simulink model "FCHEV_sideRadiator"  (R2023a)
settings: Solver=ode23tb  StartTime=0.0  StopTime=20e3  MaxStep=1  RelTol=1e-3
values from neighbouring files (symbols this model uses):
  fc_current = 170    [run_FCHEV_simulations.m]
  mass = 20e3    (= 20000)    [run_BEV_simulations.m]    (also in run_FCHEV_simulations.m)
libraries: component_lib x158, slpidlib x10, simulink x1
(part 1 of 2)
settings Model: Creator=maxjo65  LastModifiedBy=maxjo
settings SolverCC: ZeroCrossControl=DisableAll
settings OptimizationCC: ReuseModelBlockBuffer=off
settings DebuggingCC: UnconnectedInputMsg=warning  UnconnectedOutputMsg=warning  UnconnectedLineMsg=warning
settings ModelReferenceCC: EnableRefExpFcnMdlSchedulingChecks=on
settings RTWCC: DLArmComputeVersion=19.05

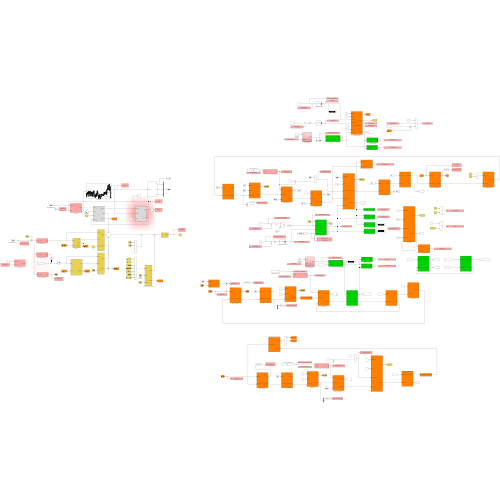
[thumbnail: Simulink's stored preview of the top-level diagram]
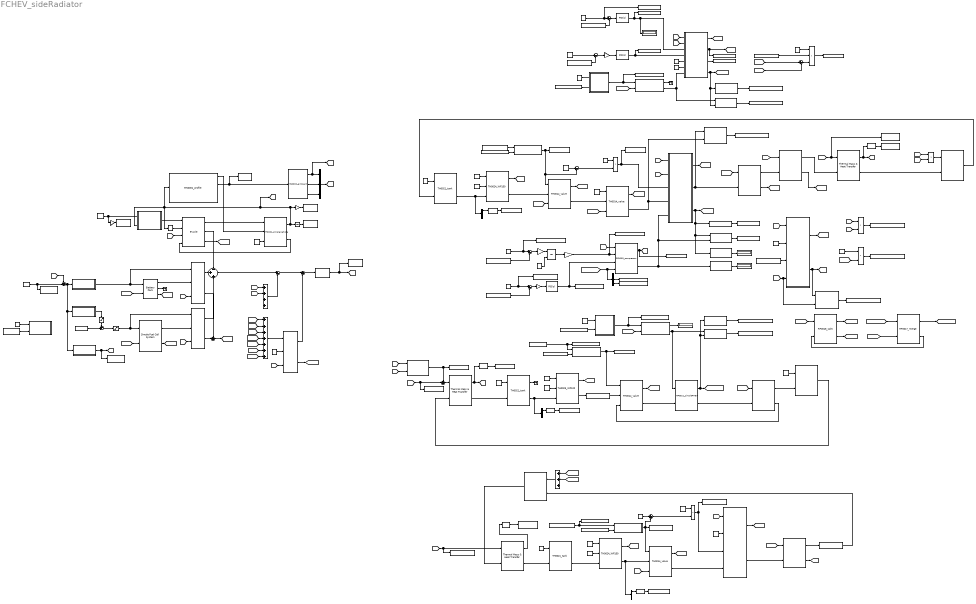
== system FCHEV_sideRadiator ==
  Add Constant{,1..5} (6 alike) : Bias  Bias=-273.15  SaturateOnIntegerOverflow=off
  Add1 : Sum  Inputs=++++
  Add2 : Sum  Inputs=+++++++
  Add3 : Sum  Inputs=+++
  Battery : component_lib/Battery Pack  SOC_0=0.5  Nx=120  Ny=125
  Battery Heater : component_lib/Thermal Systems/TH0015_totalHeatTransfer  T_max=273+100  T_min=273
  Battery Heater1 : component_lib/Thermal Systems/TH0015_totalHeatTransfer  T_max=273+100  T_min=273
  Battery Thermal Mass : component_lib/Thermal Mass & Heat Transfer  n=100  d=10e-3  L=4  m=120 * 125 * 0.048  cp=1040  T_0=273 + 26
  Bus Voltage Control 1 : Subsystem
  "Bus Voltage Control 2 " : Subsystem
  Bus Voltage Control 3 : Subsystem
  Bus Voltage Reference [V] : Constant  Value=700
  Cabin Airflow Controller : slpidlib/PID Controller  Controller=PID  Form=Parallel  TimeDomain=Continuous-time  UseExternalTs=off  SampleTime=-1  IntegratorMethod=Forward Euler  FilterMethod=Forward Euler  ControllerParametersSource=internal  P=1  I=1e-1  UseKiTs=off  D=0  N=100  UseFilter=on  TunerSelectOption=Transfer Function Based (PID Tuner App)  InitialConditionSource=internal  InitialConditionForIntegrator=0.5  InitialConditionForFilter=0.5  DifferentiatorICPrevScaledInput=0  ExternalReset=none  TrackingMode=off  Kt=1  LimitOutput=on  SatLimitsSource=internal  UpperSaturationLimit=0.99  LowerSaturationLimit=0.01  LinearizeAsGain=on  AntiWindupMode=clamping  Kb=1  LimitIntegrator=off  UpperIntegratorSaturationLimit=inf  LowerIntegratorSaturationLimit=-inf  POutMin=[]  POutMax=[]  IOutMin=[]  IOutMax=[]  DOutMin=[]  DOutMax=[]  NOutMin=[]  NOutMax=[]  SumOutMin=[]  SumOutMax=[]  SaturationOutMin=[]  SaturationOutMax=[]  PParamMin=[]  PParamMax=[]  IParamMin=[]  IParamMax=[]  DParamMin=[]  DParamMax=[]  NParamMin=[]  NParamMax=[]  KbParamMin=[]  KbParamMax=[]  KtParamMin=[]  KtParamMax=[]  KbOutMin=[]  KbOutMax=[]  KtOutMin=[]  KtOutMax=[]  IntegratorOutMin=[]  IntegratorOutMax=[]  FilterOutMin=[]  FilterOutMax=[]  SumI1OutMin=[]  SumI1OutMax=[]  SumI2OutMin=[]  SumI2OutMax=[]  SumI3OutMin=[]  SumI3OutMax=[]  SumI4OutMin=[]  SumI4OutMax=[]  SumDOutMin=[]  SumDOutMax=[]  DifferentiatorOutMin=[]  DifferentiatorOutMax=[]  FilterDiffOutCoefMin=[]  FilterDiffOutCoefMax=[]  ReciprocalOutMin=[]  ReciprocalOutMax=[]  SumDenOutMin=[]  SumDenOutMax=[]  SumNumOutMin=[]  SumNumOutMax=[]  DivideOutMin=[]  DivideOutMax=[]  UdiffTsProdOutMin=[]  UdiffTsProdOutMax=[]  NTsProdOutMin=[]  NTsProdOutMax=[]  UintegralTsProdOutMin=[]  UintegralTsProdOutMax=[]  UngainTsProdOutMin=[]  UngainTsProdOutMax=[]  ClampingZeroOutDataTypeStr=Inherit: Inherit via back propagation  ClampingZeroOutMin=[]  ClampingZeroOutMax=[]  FilterDenConstantOutDataTypeStr=Inherit: Inherit via back propagation  FilterDenConstantOutMin=[]  FilterDenConstantOutMax=[]  PCopyOutDataTypeStr=Inherit: Inherit via back propagation  PCopyOutMin=[]  PCopyOutMax=[]  NCopyOutDataTypeStr=Inherit: Inherit via back propagation  NCopyOutMin=[]  NCopyOutMax=[]  IntegratorContinuousStateAttributes=''  IntegratorStateMustResolveToSignalObject=off  IntegratorRTWStateStorageClass=Auto  FilterContinuousStateAttributes=''  FilterStateMustResolveToSignalObject=off  FilterRTWStateStorageClass=Auto  ParallelPVariant=InternalParameters  IdealPVariant=Disabled  IVariant=InternalParameters  DVariant=InternalParameters  IntegratorVariant=Continuous  SatVariant=Enabled  AWVariant=ContClampingParallel  PCopyVariant=Disabled  TRVariant=Disabled  FdbkBlocksVariant=Forward  IdealPFdbkVariant=Disabled  SatFdbkVariant=Disabled  DerivativeFilterVariant=ContFilter  NVariant=InternalParameters  NCopyVariant=Disabled  FilterICVariant=InternalICsFilter  IntegratorICVariant=InternalICs  ExternalResetVariant=Disabled  TRSumVariant=Passthrough  SumFdbkVariant=Disabled  SumVariant=Sum_PID  TsampFilterVariant=InternalTs  TsampNgainVariant=Passthrough  TsampIntegralVariant=Disabled_SignalSpec  ExternalSaturationOutDataTypeStr=Inherit: Same as second input
  Cabin Temperature Controller : slpidlib/PID Controller  Controller=PID  Form=Parallel  TimeDomain=Continuous-time  UseExternalTs=off  SampleTime=-1  IntegratorMethod=Forward Euler  FilterMethod=Forward Euler  ControllerParametersSource=internal  P=1e-1  I=1e-2  UseKiTs=off  D=0  N=100  UseFilter=on  TunerSelectOption=Transfer Function Based (PID Tuner App)  InitialConditionSource=internal  InitialConditionForIntegrator=0.5  InitialConditionForFilter=0.5  DifferentiatorICPrevScaledInput=0  ExternalReset=none  TrackingMode=off  Kt=1  LimitOutput=on  SatLimitsSource=internal  UpperSaturationLimit=0.99  LowerSaturationLimit=0.01  LinearizeAsGain=on  AntiWindupMode=clamping  Kb=1  LimitIntegrator=off  UpperIntegratorSaturationLimit=inf  LowerIntegratorSaturationLimit=-inf  POutMin=[]  POutMax=[]  IOutMin=[]  IOutMax=[]  DOutMin=[]  DOutMax=[]  NOutMin=[]  NOutMax=[]  SumOutMin=[]  SumOutMax=[]  SaturationOutMin=[]  SaturationOutMax=[]  PParamMin=[]  PParamMax=[]  IParamMin=[]  IParamMax=[]  DParamMin=[]  DParamMax=[]  NParamMin=[]  NParamMax=[]  KbParamMin=[]  KbParamMax=[]  KtParamMin=[]  KtParamMax=[]  KbOutMin=[]  KbOutMax=[]  KtOutMin=[]  KtOutMax=[]  IntegratorOutMin=[]  IntegratorOutMax=[]  FilterOutMin=[]  FilterOutMax=[]  SumI1OutMin=[]  SumI1OutMax=[]  SumI2OutMin=[]  SumI2OutMax=[]  SumI3OutMin=[]  SumI3OutMax=[]  SumI4OutMin=[]  SumI4OutMax=[]  SumDOutMin=[]  SumDOutMax=[]  DifferentiatorOutMin=[]  DifferentiatorOutMax=[]  FilterDiffOutCoefMin=[]  FilterDiffOutCoefMax=[]  ReciprocalOutMin=[]  ReciprocalOutMax=[]  SumDenOutMin=[]  SumDenOutMax=[]  SumNumOutMin=[]  SumNumOutMax=[]  DivideOutMin=[]  DivideOutMax=[]  UdiffTsProdOutMin=[]  UdiffTsProdOutMax=[]  NTsProdOutMin=[]  NTsProdOutMax=[]  UintegralTsProdOutMin=[]  UintegralTsProdOutMax=[]  UngainTsProdOutMin=[]  UngainTsProdOutMax=[]  ClampingZeroOutDataTypeStr=Inherit: Inherit via back propagation  ClampingZeroOutMin=[]  ClampingZeroOutMax=[]  FilterDenConstantOutDataTypeStr=Inherit: Inherit via back propagation  FilterDenConstantOutMin=[]  FilterDenConstantOutMax=[]  PCopyOutDataTypeStr=Inherit: Inherit via back propagation  PCopyOutMin=[]  PCopyOutMax=[]  NCopyOutDataTypeStr=Inherit: Inherit via back propagation  NCopyOutMin=[]  NCopyOutMax=[]  IntegratorContinuousStateAttributes=''  IntegratorStateMustResolveToSignalObject=off  IntegratorRTWStateStorageClass=Auto  FilterContinuousStateAttributes=''  FilterStateMustResolveToSignalObject=off  FilterRTWStateStorageClass=Auto  ParallelPVariant=InternalParameters  IdealPVariant=Disabled  IVariant=InternalParameters  DVariant=InternalParameters  IntegratorVariant=Continuous  SatVariant=Enabled  AWVariant=ContClampingParallel  PCopyVariant=Disabled  TRVariant=Disabled  FdbkBlocksVariant=Forward  IdealPFdbkVariant=Disabled  SatFdbkVariant=Disabled  DerivativeFilterVariant=ContFilter  NVariant=InternalParameters  NCopyVariant=Disabled  FilterICVariant=InternalICsFilter  IntegratorICVariant=InternalICs  ExternalResetVariant=Disabled  TRSumVariant=Passthrough  SumFdbkVariant=Disabled  SumVariant=Sum_PID  TsampFilterVariant=InternalTs  TsampNgainVariant=Passthrough  TsampIntegralVariant=Disabled_SignalSpec  ExternalSaturationOutDataTypeStr=Inherit: Same as second input
  Cabin with Evaporator : Subsystem
  Calculate Superheat1 : component_lib/Thermal Systems/RF0010_calculateSuperHeat
  Calculate Superheat2 : component_lib/Thermal Systems/RF0010_calculateSuperHeat
  Chassi : component_lib/Powertrain/PT0001_simpleVehicle  m=mass  r_w=0.5  A_f=10  C_d=0.5  rho_air=1.225  c_r0=0.0060  c_r1=2.3e-7  gain=600  v0=80/3.6  x0=0
  Chiller Bypass : component_lib/Thermal Systems/TH0014_valve  d=10e-2  dr=5e-2  C_d=0.9
  Compressor Speed Controller : slpidlib/PID Controller  Controller=PID  Form=Parallel  TimeDomain=Continuous-time  UseExternalTs=off  SampleTime=-1  IntegratorMethod=Forward Euler  FilterMethod=Forward Euler  ControllerParametersSource=internal  P=1e2  I=1e1  UseKiTs=off  D=0  N=100  UseFilter=on  TunerSelectOption=Transfer Function Based (PID Tuner App)  InitialConditionSource=internal  InitialConditionForIntegrator=2000  InitialConditionForFilter=2000  DifferentiatorICPrevScaledInput=0  ExternalReset=none  TrackingMode=off  Kt=1  LimitOutput=on  SatLimitsSource=internal  UpperSaturationLimit=5000  LowerSaturationLimit=100  LinearizeAsGain=on  AntiWindupMode=clamping  Kb=1  LimitIntegrator=off  UpperIntegratorSaturationLimit=inf  LowerIntegratorSaturationLimit=-inf  POutMin=[]  POutMax=[]  IOutMin=[]  IOutMax=[]  DOutMin=[]  DOutMax=[]  NOutMin=[]  NOutMax=[]  SumOutMin=[]  SumOutMax=[]  SaturationOutMin=[]  SaturationOutMax=[]  PParamMin=[]  PParamMax=[]  IParamMin=[]  IParamMax=[]  DParamMin=[]  DParamMax=[]  NParamMin=[]  NParamMax=[]  KbParamMin=[]  KbParamMax=[]  KtParamMin=[]  KtParamMax=[]  KbOutMin=[]  KbOutMax=[]  KtOutMin=[]  KtOutMax=[]  IntegratorOutMin=[]  IntegratorOutMax=[]  FilterOutMin=[]  FilterOutMax=[]  SumI1OutMin=[]  SumI1OutMax=[]  SumI2OutMin=[]  SumI2OutMax=[]  SumI3OutMin=[]  SumI3OutMax=[]  SumI4OutMin=[]  SumI4OutMax=[]  SumDOutMin=[]  SumDOutMax=[]  DifferentiatorOutMin=[]  DifferentiatorOutMax=[]  FilterDiffOutCoefMin=[]  FilterDiffOutCoefMax=[]  ReciprocalOutMin=[]  ReciprocalOutMax=[]  SumDenOutMin=[]  SumDenOutMax=[]  SumNumOutMin=[]  SumNumOutMax=[]  DivideOutMin=[]  DivideOutMax=[]  UdiffTsProdOutMin=[]  UdiffTsProdOutMax=[]  NTsProdOutMin=[]  NTsProdOutMax=[]  UintegralTsProdOutMin=[]  UintegralTsProdOutMax=[]  UngainTsProdOutMin=[]  UngainTsProdOutMax=[]  ClampingZeroOutDataTypeStr=Inherit: Inherit via back propagation  ClampingZeroOutMin=[]  ClampingZeroOutMax=[]  FilterDenConstantOutDataTypeStr=Inherit: Inherit via back propagation  FilterDenConstantOutMin=[]  FilterDenConstantOutMax=[]  PCopyOutDataTypeStr=Inherit: Inherit via back propagation  PCopyOutMin=[]  PCopyOutMax=[]  NCopyOutDataTypeStr=Inherit: Inherit via back propagation  NCopyOutMin=[]  NCopyOutMax=[]  IntegratorContinuousStateAttributes=''  IntegratorStateMustResolveToSignalObject=off  IntegratorRTWStateStorageClass=Auto  FilterContinuousStateAttributes=''  FilterStateMustResolveToSignalObject=off  FilterRTWStateStorageClass=Auto  ParallelPVariant=InternalParameters  IdealPVariant=Disabled  IVariant=InternalParameters  DVariant=InternalParameters  IntegratorVariant=Continuous  SatVariant=Enabled  AWVariant=ContClampingParallel  PCopyVariant=Disabled  TRVariant=Disabled  FdbkBlocksVariant=Forward  IdealPFdbkVariant=Disabled  SatFdbkVariant=Disabled  DerivativeFilterVariant=ContFilter  NVariant=InternalParameters  NCopyVariant=Disabled  FilterICVariant=InternalICsFilter  IntegratorICVariant=InternalICs  ExternalResetVariant=Disabled  TRSumVariant=Passthrough  SumFdbkVariant=Disabled  SumVariant=Sum_PID  TsampFilterVariant=InternalTs  TsampNgainVariant=Passthrough  TsampIntegralVariant=Disabled_SignalSpec  ExternalSaturationOutDataTypeStr=Inherit: Same as second input
  Constant : Constant  Value=0.3
  Constant{1,11,13,19,27} (5 alike) : Constant  Value=0
  Constant{6,8,10,17} (4 alike) : Constant  Value=24
  Constant12 : Constant  Value=23
  Constant14 : Constant  Value=0.1
  Constant15 : Constant  Value=2e5
  Constant16 : Constant  Value=4000
  Constant{2,5,18,21,26} (5 alike) : Constant  Value=3000
  Constant20 : Constant  Value=22.5
  Constant23 : Constant  Value=10
  Constant24 : Constant  Value=15
  Constant25 : Constant
  Constant28 : Constant
  Constant3 : Constant  Value=0.5
  Constant4 : Constant  Value=2e5
  Constant7 : Constant  Value=2e5
  Constant9 : Constant  Value=fc_current
  DC/DC - Low level converter : component_lib/Electrochemistry/EL0008_dcdcConverter  eta_up=0.98  eta_down=0.98
  DC/DC Converter : component_lib/Electrochemistry/EL0008_dcdcConverter  eta_up=0.99  eta_down=0.99
  DC/DC Converter1 : component_lib/Electrochemistry/EL0008_dcdcConverter  eta_up=0.99  eta_down=0.99
  Demux{,1..3} (4 alike) : Demux  Outputs=3
  Display{,1..3} (4 alike) : Display
  Fuel Cell Thermal Mass : component_lib/Thermal Mass & Heat Transfer  n=375*2*20  d=2e-3  L=50e-2  m=72  cp=420  T_0=273 + 80
  Gain : Gain  Gain=3.6
  Gain1 : Gain  Gain=3.6
  Gain2 : Gain  Gain=-1
  Gain3 : Gain  Gain=-1
  Gain4 : Gain  Gain=1e5
  Gain5 : Gain  Gain=1e-1
  Gear selector : Relay  OnSwitchValue=22  OffSwitchValue=21.5  OnOutputValue=4  OffOutputValue=3
  Integrator : Integrator
  Integrator1 : Integrator  InitialConditionSource=external  LimitOutput=on  UpperSaturationLimit=30  LowerSaturationLimit=8
  Low Voltage Bus Level : Constant  Value=24
  MN0002_ambient : component_lib/Mission/MN0002_ambient  p_0=1.01e5  T_0=T_amb  RH_0=0.2
  Motor Heat Transfer : component_lib/Thermal Mass & Heat Transfer  n=100*3  d=5e-3  L=30e-2  m=200  cp=420  T_0=273 + 70
  Motor Temperature Reference : Constant  Value=70
  Motor and Gearbox : component_lib/E-Axle  n=4  V_nom=700
  Mux : Mux  Inputs=3
  Power Electronics Heat Transfer : component_lib/Thermal Systems/TH0015_totalHeatTransfer  T_max=273+100  T_min=273
  Product : Product  Inputs=***
  Product{1..5} (5 alike) : Product
  RF0003_compressor : component_lib/Thermal Systems/RF0003_compressor  V_disp=0.00017  N_ref=2000  t_c=1  W0=25e-3
  RF0011_calculateSubCool : component_lib/Thermal Systems/RF0011_calculateSubCool
  RF0013_calculateHeatflow1 : component_lib/Thermal Systems/RF0013_calculateHeatflow
  RF0013_calculateHeatflow2 : component_lib/Thermal Systems/RF0013_calculateHeatflow
  RF0013_calculateHeatflow3 : component_lib/Thermal Systems/RF0013_calculateHeatflow
  RF0016_split : component_lib/Thermal Systems/RF0016_split
  RF0017_merge : component_lib/Thermal Systems/RF0017_merge  V=1e-3
  RF0018_calculateTemperature : component_lib/Thermal Systems/RF0018_calculateTemperature
  RF0018_calculateTemperature1 : component_lib/Thermal Systems/RF0018_calculateTemperature
  RF0021_simplePHEX : component_lib/Thermal Systems/RF0021_simplePHEX  N_ch=10  L=180e-3  B=65e-3  H=2e-3  t=0.3e-3  D_h=2.61e-3
  RF0022_simpleExpansionValve : component_lib/Thermal Systems/RF0022_simpleExpansionValve  D=4*1.8e-3  p_min=100e3  C=0.3
  RF0022_simpleExpansionValve1 : component_lib/Thermal Systems/RF0022_simpleExpansionValve  D=4*1.8e-3  p_min=100e3  C=0.3
  Radiator & Condenser Assembly : Subsystem
  Radiator Bypass Valve : component_lib/Thermal Systems/TH0014_valve  d=10e-2  dr=5e-2  C_d=0.9
  Radiator Bypass Valve1 : component_lib/Thermal Systems/TH0014_valve  d=10e-2  dr=5e-2  C_d=0.9
  Road Profile : component_lib/Mission/MN0001_profile  profile=Sodertalje_Norrkoping.mat  x0=0  N_lookahead=100
  SC0002_signalRead : component_lib/Data & Control/SC0002_signalRead  SigName=velocity
  SC0002_signalRead1 : component_lib/Data & Control/SC0002_signalRead  SigName=condenserCooling
  SC0002_signalRead10 : component_lib/Data & Control/SC0002_signalRead  SigName=condenserSubcool
  SC0002_signalRead11 : component_lib/Data & Control/SC0002_signalRead  SigName=chillerBypassValve
  SC0002_signalRead12 : component_lib/Data & Control/SC0002_signalRead  SigName=batteryTemperatureReference
  SC0002_signalRead13 : component_lib/Data & Control/SC0002_signalRead  SigName=cabinFreshAirFlowReference
  SC0002_signalRead14 : component_lib/Data & Control/SC0002_signalRead  SigName=intakeFlap
  SC0002_signalRead15 : component_lib/Data & Control/SC0002_signalRead  SigName=cabinFreshAirFlow
  SC0002_signalRead16 : component_lib/Data & Control/SC0002_signalRead  SigName=batteryConvection
  SC0002_signalRead17 : component_lib/Data & Control/SC0002_signalRead  SigName=batteryCoolantTemperature
  SC0002_signalRead18 : component_lib/Data & Control/SC0002_signalRead  SigName=fuelCellTemperature
  SC0002_signalRead19 : component_lib/Data & Control/SC0002_signalRead  SigName=radiatorBypassValve
  SC0002_signalRead2 : component_lib/Data & Control/SC0002_signalRead  SigName=altitude
  SC0002_signalRead20 : component_lib/Data & Control/SC0002_signalRead  SigName=evaporatorExpansionValve
  SC0002_signalRead21 : component_lib/Data & Control/SC0002_signalRead  SigName=mainRadiatorFanSpeed
  SC0002_signalRead22 : component_lib/Data & Control/SC0002_signalRead  SigName=batteryTemperature
  SC0002_signalRead23 : component_lib/Data & Control/SC0002_signalRead  SigName=evaporatorSuperheat
  SC0002_signalRead24 : component_lib/Data & Control/SC0002_signalRead  SigName=chillerCooling
  SC0002_signalRead25 : component_lib/Data & Control/SC0002_signalRead  SigName=motorTemperature
  SC0002_signalRead26 : component_lib/Data & Control/SC0002_signalRead  SigName=sideRadiatorBypassValve
  SC0002_signalRead27 : component_lib/Data & Control/SC0002_signalRead  SigName=motorCoolantTemperatureReference
  SC0002_signalRead28 : component_lib/Data & Control/SC0002_signalRead  SigName=chillerSuperheat
  SC0002_signalRead29 : component_lib/Data & Control/SC0002_signalRead  SigName=cabinFanCurrent
  SC0002_signalRead3 : component_lib/Data & Control/SC0002_signalRead  SigName=velocityReference
  SC0002_signalRead30 : component_lib/Data & Control/SC0002_signalRead  SigName=chillerExpansionValve
  SC0002_signalRead31 : component_lib/Data & Control/SC0002_signalRead  SigName=evaporatorCooling
  SC0002_signalRead33 : component_lib/Data & Control/SC0002_signalRead  SigName=evaporatorFlap
  SC0002_signalRead34 : component_lib/Data & Control/SC0002_signalRead  SigName=compressorCurrent
  SC0002_signalRead35 : component_lib/Data & Control/SC0002_signalRead  SigName=condenserPressure
  SC0002_signalRead36 : component_lib/Data & Control/SC0002_signalRead  SigName=fuelCellLosses
  SC0002_signalRead37 : component_lib/Data & Control/SC0002_signalRead  SigName=fanPower
  SC0002_signalRead38 : component_lib/Data & Control/SC0002_signalRead  SigName=evaporatorPressure
  SC0002_signalRead39 : component_lib/Data & Control/SC0002_signalRead  SigName=compressorFlow
  SC0002_signalRead4 : component_lib/Data & Control/SC0002_signalRead  SigName=busVoltage
  SC0002_signalRead40 : component_lib/Data & Control/SC0002_signalRead  SigName=compressorPower
  SC0002_signalRead41 : component_lib/Data & Control/SC0002_signalRead  SigName=batteryLosses
  SC0002_signalRead42 : component_lib/Data & Control/SC0002_signalRead  SigName=cabinIntakeHeat
  SC0002_signalRead43 : component_lib/Data & Control/SC0002_signalRead  SigName=condenserSubcoolReference
  SC0002_signalRead44 : component_lib/Data & Control/SC0002_signalRead  SigName=sideRadiatorCooling
  SC0002_signalRead45 : component_lib/Data & Control/SC0002_signalRead  SigName=mainRadiatorCooling
  SC0002_signalRead46 : component_lib/Data & Control/SC0002_signalRead  SigName=motorLosses
  SC0002_signalRead47 : component_lib/Data & Control/SC0002_signalRead  SigName=motorRadiatorFanSpeed
  SC0002_signalRead48 : component_lib/Data & Control/SC0002_signalRead  SigName=compressorSpeed
  SC0002_signalRead49 : component_lib/Data & Control/SC0002_signalRead  SigName=cabinTemperatureReference
  SC0002_signalRead5 : component_lib/Data & Control/SC0002_signalRead  SigName=distance
  SC0002_signalRead6 : component_lib/Data & Control/SC0002_signalRead  SigName=busVoltageReference
  SC0002_signalRead7 : component_lib/Data & Control/SC0002_signalRead  SigName=burnoffCurrent
  SC0002_signalRead8 : component_lib/Data & Control/SC0002_signalRead  SigName=fuelCellCoolantTemperature
  SC0002_signalRead9 : component_lib/Data & Control/SC0002_signalRead  SigName=motorCoolantTemperature
  SC0003_signalWrite : component_lib/Data & Control/SC0003_signalWrite  SigName=stateOfCharge
  SC0003_signalWrite1 : component_lib/Data & Control/SC0003_signalWrite  SigName=batteryCoolantTemperature
  SC0003_signalWrite10 : component_lib/Data & Control/SC0003_signalWrite  SigName=mainRadiatorFanSpeed
  SC0003_signalWrite15 : component_lib/Data & Control/SC0003_signalWrite  SigName=cabinFreshAirFlow
  SC0003_signalWrite2 : component_lib/Data & Control/SC0003_signalWrite  SigName=cabinFreshAirFlow
  SC0003_signalWrite3 : component_lib/Data & Control/SC0003_signalWrite  SigName=fuelCellTemperature
  SC0003_signalWrite4 : component_lib/Data & Control/SC0003_signalWrite  SigName=motorCoolantTemperature
  SC0003_signalWrite5 : component_lib/Data & Control/SC0003_signalWrite  SigName=chillerSuperheat
  SC0003_signalWrite6 : component_lib/Data & Control/SC0003_signalWrite  SigName=evaporatorSuperheat
  SC0003_signalWrite7 : component_lib/Data & Control/SC0003_signalWrite  SigName=cabinTemperature
  SC0003_signalWrite8 : component_lib/Data & Control/SC0003_signalWrite  SigName=cabinTemperature
  SC0003_signalWrite9 : component_lib/Data & Control/SC0003_signalWrite  SigName=condenserSubcool
  SOC-reference : Subsystem
  Saturation : Saturate  UpperLimit=500  LowerLimit=20
  Saturation1 : Saturate  UpperLimit=0  LowerLimit=-inf
  Side Radiator Valve : component_lib/Thermal Systems/TH0014_valve  d=10e-2  dr=5e-2  C_d=0.9
  Side radiator : Subsystem  mask{HtH=0.5, StS=0.5}
      mask prompts: HtH "Header to header [m]"; StS "Sideplate to sideplate [m]"
  Simple Fuel Cell System : component_lib/Simple Fuel Cell System  n_st=2  n=400
  Single Air Stream Heat Exchanger : Subsystem  mask{HtH=0.5, StS=0.5}
      mask prompts: HtH "Header to header [m]"; StS "Sideplate to sideplate [m]"
  Speed control : Subsystem
  Speed reference [m/s] : Constant  Value=80/3.6
  Subsystem1 : Subsystem
  Subsystem2 : Subsystem
  Subsystem4 : Subsystem
  Sum : Sum  Inputs=-++
  Sum1 : Sum  Inputs=-+|
  Sum{3..4,7..13} (9 alike) : Sum  Inputs=|+-
  Sum2 : Sum  Inputs=++|
  Sum5 : Sum  Inputs=++|
  Sum6 : Sum  Inputs=++|
  Super Capacitor : component_lib/Electrochemistry/EL0010_superCapacitor  C=1  V_bus0=700
  Superheat Control : Subsystem
  Superheat Control1 : Subsystem
  Superheating Reference : Constant  Value=5
  Superheating Reference1 : Constant  Value=5
  TH0006_flowConfluence{1..4} (4 alike) : component_lib/Thermal Systems/TH0006_flowConfluence  gain=0.01
  TH0011_pipe1 : component_lib/Thermal Systems/TH0011_pipe  d=19e-3  L=2  e=0.006e-3  T_0=273 + 20
  TH0011_pipe2 : component_lib/Thermal Systems/TH0011_pipe  d=32e-3  L=2  e=0.006e-3  T_0=273 + 20
  TH0016_calculateHeatflow : component_lib/Thermal Systems/TH0016_calculateHeatflow
  TH0016_calculateHeatflow1 : component_lib/Thermal Systems/TH0016_calculateHeatflow
  TH0021_tank : component_lib/Thermal Systems/TH0021_tank  V=5e-3  T0=273.15 + 25
  TH0021_tank1 : component_lib/Thermal Systems/TH0021_tank  V=5e-3  T0=273.15 + 80
  TH0021_tank2 : component_lib/Thermal Systems/TH0021_tank  V=5e-3  T0=273.15 + 70
  TH0023_WP120 : component_lib/Thermal Systems/TH0023_WP120  SystemSampleTime=-1  VariantActivationTime=update diagram  Latency=0  AutoFrameSizeCalculation=off
  TH0024_WP1 : component_lib/Thermal Systems/TH0024_WP150  n=2
      settings: LibrarySourceBlock=component_lib/Thermal Systems/TH0023_WP120
  TH0024_WP150 : component_lib/Thermal Systems/TH0024_WP150  n=2
      settings: LibrarySourceBlock=component_lib/Thermal Systems/TH0023_WP120
  TH0030_batteryPackConvection : component_lib/Thermal Systems/TH0030_batteryPackConvection  A=2*10  h=8
  Temperature Reference : Constant  Value=80
  Temperature Reference2 : Constant  Value=25
  Terminator : Terminator
  Terminator2 : Terminator
  Terminator3 : Terminator
  cp_air : Constant  Value=1e3
  wires:
  Motor and Gearbox/1 -> Chassi/1
  Chassi/2 -> Motor and Gearbox/4
  Road Profile/1 -> Chassi/2
  Chassi/1 -> Integrator/1, Gain/1, [v], Speed control/2(v [m/s]), Road Profile/1, Gear selector/1
  Speed reference [m/s]/1 -> Gain1/1, Speed control/1(v_ref [m/s])
  Speed control/1(Tq_sig [-]) -> Motor and Gearbox/1
  Gear selector/1 -> Motor and Gearbox/2
  Integrator/1 -> SC0002_signalRead5/1
  Gain/1 -> SC0002_signalRead/1
  Road Profile/2 -> MN0002_ambient/1, SC0002_signalRead2/1
  Gain1/1 -> SC0002_signalRead3/1
  Super Capacitor/1 -> SC0002_signalRead4/1, [V_bus]
  Constant1/1 -> Chassi/3
  Battery/1 -> DC/DC Converter/2
  DC/DC Converter/1 -> Sum/2
  Motor and Gearbox/2 -> Sum/1
  Bus Voltage Control 1/1(I_bat [-]) -> DC/DC Converter/1, Battery/1
  DC/DC Converter1/1 -> Sum/3
  Bus Voltage Reference [V]/1 -> Sum1/2, SC0002_signalRead6/1
  Constant3/1 -> SOC-reference/1(SOC_ref [-])
  SC0003_signalWrite/1 -> SOC-reference/2(SOC [-])
  Sum1/1 -> Bus Voltage Control 3/1(V_ref - V_bus [V]), "Bus Voltage Control 2 "/1(V_ref - V_bus [V]), Bus Voltage Control 1/1(V_ref - V_bus [V])
  Sum2/1 -> Saturation/1
  Sum/1 -> Sum3/1
  Bus Voltage Control 3/1(I_bf [A]) -> SC0002_signalRead7/1, [I_bf]
  Simple Fuel Cell System/1 -> DC/DC Converter1/2
  Sum3/1 -> Sum4/1
  Saturation/1 -> DC/DC Converter1/1, Simple Fuel Cell System/1
  [T_bat] -> Battery/2
  Sum4/1 -> Super Capacitor/1
  Low Voltage Bus Level/1 -> DC/DC - Low level converter/2
  DC/DC - Low level converter/1 -> Sum4/2
  DC/DC - Low level converter/2 -> [Q_LVDCDC]
  [I_cabFan] -> Add2/1
  [I_batPump] -> Add2/2
  [V_bus] -> DC/DC - Low level converter/3
  [I_radPump] -> Add2/3
  Add2/1 -> DC/DC - Low level converter/1
  Sum5/1 -> Battery Thermal Mass/1
  [T_bat] -> TH0030_batteryPackConvection/2
  TH0021_tank/2 -> Demux/1, TH0023_WP120/3
  TH0023_WP120/1 -> [I_batPump]
  Add Constant1/1 -> SC0002_signalRead17/1
  Constant6/1 -> TH0023_WP120/1
  TH0021_tank/1 -> Terminator3/1
  Add Constant/1 -> SC0002_signalRead22/1
  RF0021_simplePHEX/1 -> Calculate Superheat1/1, RF0013_calculateHeatflow1/2, [RF_CHILLER_OUT]
  TH0011_pipe1/1 -> Chiller Bypass/2
  TH0030_batteryPackConvection/1 -> Sum5/1, SC0002_signalRead16/1
  RF0022_simpleExpansionValve/2 -> RF0021_simplePHEX/1, RF0013_calculateHeatflow1/1
  Constant5/1 -> TH0023_WP120/2
  Demux/1 -> Add Constant1/1
  Constant4/1 -> TH0021_tank/1
  RF0013_calculateHeatflow1/1 -> SC0002_signalRead24/1
  Battery Thermal Mass/2 -> TH0021_tank/2
  Battery Thermal Mass/1 -> [T_bat], Add Constant/1
  TH0023_WP120/2 -> TH0011_pipe1/1
  [T_amb] -> TH0030_batteryPackConvection/1
  MN0002_ambient/2 -> Mux/2
  MN0002_ambient/3 -> Mux/3
  MN0002_ambient/1 -> [T_amb], Mux/1
  Mux/1 -> [amb]
  Simple Fuel Cell System/2 -> [Q_fc]
  Battery/3 -> [Q_bat]
  Motor and Gearbox/3 -> [Q_em]
  DC/DC Converter1/2 -> Sum6/2
  Sum6/1 -> [Q_HVDCDC]
  DC/DC Converter/2 -> Sum6/1
  [T_fc] -> Simple Fuel Cell System/2
  [V_bus] -> Motor and Gearbox/3
  [V_bus] -> Sum1/1
  [V_bus] -> DC/DC Converter/3
  [V_bus] -> DC/DC Converter1/3
  Superheating Reference/1 -> Superheat Control/1(T_ref [K])
  [RF_CHILLER_IN] -> RF0022_simpleExpansionValve/2
  SC0003_signalWrite5/1 -> Superheat Control/2(T_sup [K])
  Superheat Control/1(EXV [-]) -> RF0022_simpleExpansionValve/1, SC0002_signalRead30/1
  RF0022_simpleExpansionValve/1 -> Display/1
  Radiator Bypass Valve/1 -> [CL1]
  Battery Heater1/1 -> TH0021_tank1/2
  Temperature Reference/1 -> Subsystem1/1(T_ref [K])
  Radiator & Condenser Assembly/2(CL: (T2,p2,W2)) -> TH0016_calculateHeatflow1/1, TH0006_flowConfluence1/2
  Constant7/1 -> TH0021_tank1/1
  [Q_fc] -> SC0002_signalRead36/1, Fuel Cell Thermal Mass/1
  SC0003_signalWrite3/1 -> Subsystem1/2(T_fc [K])
  Radiator Bypass Valve/2 -> Side Radiator Valve/2
  Fuel Cell Thermal Mass/1 -> [T_fc], Add Constant2/1
  [v] -> Radiator & Condenser Assembly/2(v [m/s])
  [amb] -> Radiator & Condenser Assembly/1(AMB: (T,p,RH))
  Radiator & Condenser Assembly/1(I_fan [A]) -> [I_radFan]
  Radiator & Condenser Assembly/3(RF: (h2,p2,W2)) -> RF0018_calculateTemperature/1, RF0013_calculateHeatflow2/1, RF0011_calculateSubCool/1, [RF_COND_OUT]
  RF0003_compressor/2 -> RF0013_calculateHeatflow2/2, Radiator & Condenser Assembly/5(RF: (h1,p1,W1)), RF0018_calculateTemperature1/1
  [I_bf] -> Add1/1
  Add1/1 -> Sum3/2
  [I_cmp] -> Add1/2
  [V_bus] -> RF0003_compressor/1
  RF0011_calculateSubCool/1 -> SC0002_signalRead10/1
  Calculate Superheat1/1 -> SC0002_signalRead28/1
  RF0003_compressor/1 -> SC0002_signalRead34/1, [I_cmp]
  Constant2/1 -> TH0024_WP150/2
  Constant10/1 -> TH0024_WP150/1
  TH0024_WP150/1 -> [I_radPump]
  Battery/2 -> Terminator/1
  Add Constant2/1 -> SC0002_signalRead18/1
  RF0013_calculateHeatflow2/1 -> SC0002_signalRead1/1
  Chiller Bypass/2 -> RF0021_simplePHEX/2
  Subsystem4/1(cv [-]) -> Chiller Bypass/1, SC0002_signalRead11/1
  Temperature Reference2/1 -> Subsystem4/1(T_ref [K]), SC0002_signalRead12/1
  SC0003_signalWrite1/1 -> Subsystem4/2(T [K])
  Chiller Bypass/1 -> [CL2]
  RF0021_simplePHEX/2 -> TH0006_flowConfluence2/2
  [CL2] -> TH0006_flowConfluence2/1
  TH0006_flowConfluence2/2 -> Chiller Bypass/3
  TH0006_flowConfluence2/1 -> Battery Heater/2
  RF0018_calculateTemperature/1 -> Display1/1
  RF0018_calculateTemperature1/1 -> Display2/1
  Product5/1 -> SC0002_signalRead47/1, Single Air Stream Heat Exchanger/3(fan_speed [rpm])
  Radiator Bypass Valve1/2 -> Single Air Stream Heat Exchanger/4(CL: (T1,p1,W1))
  [Q_LVDCDC] -> Add3/2
  Subsystem2/1(cv [-]) -> SC0002_signalRead26/1, Sum12/2, Radiator Bypass Valve1/1
  [CL3] -> TH0006_flowConfluence3/1
  [amb] -> Single Air Stream Heat Exchanger/1(AMB: (T,p,RH))
  Constant13/1 -> Single Air Stream Heat Exchanger/2(v [m/s])
  Motor Temperature Reference/1 -> SC0002_signalRead27/1, Subsystem2/1(T_ref [K])
  [split3] -> Radiator Bypass Valve1/3
  Motor Heat Transfer/2 -> TH0021_tank2/2
  Power Electronics Heat Transfer/1 -> Motor Heat Transfer/2
  Radiator Bypass Valve1/1 -> [CL3]
  Single Air Stream Heat Exchanger/1(I_fan [A]) -> [I_sideFan1]
  SC0003_signalWrite4/1 -> Subsystem2/2(T_em [K])
  [Q_em] -> SC0002_signalRead46/1, Motor Heat Transfer/1
  Constant15/1 -> TH0021_tank2/1
  TH0006_flowConfluence3/2 -> [split3]
  TH0011_pipe2/1 -> Power Electronics Heat Transfer/2
  Add3/1 -> Power Electronics Heat Transfer/1
  [Q_HVDCDC] -> Add3/1
  Single Air Stream Heat Exchanger/2(CL: (T2,p2,W2)) -> TH0006_flowConfluence3/2
  Add Constant4/1 -> SC0002_signalRead9/1
  Demux2/1 -> Add Constant4/1
  TH0024_WP1/2 -> Demux2/1, Radiator Bypass Valve1/2
  TH0021_tank2/2 -> TH0024_WP1/3
  TH0024_WP1/1 -> [I_sidePump]
  Constant18/1 -> TH0024_WP1/2
  Constant17/1 -> TH0024_WP1/1
  [I_sidePump] -> Add2/6
  Add Constant5/1 -> SC0002_signalRead25/1
  Motor Heat Transfer/1 -> Add Constant5/1
  Cabin with Evaporator/3(fresh_flow [kg/s]) -> SC0002_signalRead15/1
  Cabin with Evaporator/2(fan_current [A]) -> [I_cabFan], SC0002_signalRead29/1
  Constant16/1 -> Cabin with Evaporator/5(fan_speed [rpm])
  [v] -> Cabin with Evaporator/2(v [m/s])
  SC0003_signalWrite2/1 -> Sum7/2
  Cabin Airflow Controller/1 -> SC0002_signalRead14/1, Display3/1, Cabin with Evaporator/3(intake_flap [-])
  Constant14/1 -> Sum7/1, SC0002_signalRead13/1
  Sum7/1 -> Cabin Airflow Controller/1
  Constant19/1 -> Cabin with Evaporator/6(Q_ptc [J/s])
  Cabin with Evaporator/1(T_cabin [K]) -> [T_cab]
  [RF_COND_OUT] -> RF0016_split/1
  RF0016_split/1 -> [RF_CHILLER_IN]
  RF0016_split/2 -> [RF_EVAP_IN]
  [RF_CHILLER_OUT] -> RF0017_merge/1
  [RF_EVAP_OUT] -> RF0017_merge/2
  RF0017_merge/1 -> [RF_COMP_IN]
  RF0017_merge/2 -> RF0016_split/2
  Superheat Control1/1(EXV [-]) -> RF0022_simpleExpansionValve1/1, SC0002_signalRead20/1
  SC0003_signalWrite6/1 -> Superheat Control1/2(T_sup [K])
  [RF_EVAP_IN] -> RF0022_simpleExpansionValve1/2
  Superheating Reference1/1 -> Superheat Control1/1(T_ref [K])
  RF0022_simpleExpansionValve1/2 -> RF0013_calculateHeatflow3/1, Cabin with Evaporator/7(RF: (h1,p1,W1))
  Cabin with Evaporator/4(RF: (h2,p2,W2)) -> RF0013_calculateHeatflow3/2, Calculate Superheat2/1, [RF_EVAP_OUT]
  RF0022_simpleExpansionValve1/1 -> Terminator2/1
  [amb] -> Cabin with Evaporator/1(AMB (T,p,RH))
  Calculate Superheat2/1 -> SC0002_signalRead23/1
  RF0013_calculateHeatflow3/1 -> SC0002_signalRead31/1
  Sum9/1 -> Gain2/1
  SC0003_signalWrite7/1 -> Sum9/2
  Cabin Temperature Controller/1 -> SC0002_signalRead33/1, Cabin with Evaporator/4(evaporator_flap [-])
  Constant20/1 -> Sum9/1
  Gain2/1 -> Cabin Temperature Controller/1
  [I_sideFan1] -> Add2/4
  [I_radFan] -> Add2/5
  TH0006_flowConfluence3/1 -> TH0011_pipe2/1
  Demux3/2 -> SC0002_signalRead38/1
  Demux3/3 -> SC0002_signalRead39/1
  [RF_COMP_IN] -> Demux3/1, RF0003_compressor/4
  [I_cmp] -> Product1/2
  Product1/1 -> SC0002_signalRead40/1
  [V_bus] -> Product1/1
  [CL5] -> TH0006_flowConfluence1/1
  TH0024_WP150/2 -> Radiator Bypass Valve/2
  TH0006_flowConfluence1/2 -> [SPLIT2]
  [SPLIT1] -> Radiator Bypass Valve/3
  Battery Heater/1 -> Battery Thermal Mass/2
  [Q_bat] -> SC0002_signalRead41/1, Sum5/2
  Constant11/1 -> Battery Heater/1
  [I_radFan] -> Product2/2
  Constant8/1 -> Product2/1
  Product2/1 -> SC0002_signalRead37/1
  Sum10/1 -> Product/3
  [T_amb] -> Sum10/1
  SC0003_signalWrite15/1 -> Product/2
  cp_air/1 -> Product/1
  Product/1 -> SC0002_signalRead42/1
  [T_cab] -> Sum10/2
  Compressor Speed Controller/1 -> RF0003_compressor/3, SC0002_signalRead48/1
  Integrator1/1 -> Gain4/1
  SC0003_signalWrite9/1 -> Sum11/2
  Constant23/1 -> SC0002_signalRead43/1, Sum11/1
  Sum11/1 -> Gain5/1
  Gain4/1 -> SC0002_signalRead35/1, RF0003_compressor/2
  Constant24/1 -> Integrator1/2
  Gain5/1 -> Integrator1/1
  Constant9/1 -> Sum2/2
  TH0021_tank1/2 -> Demux1/1, TH0024_WP150/3
  Fuel Cell Thermal Mass/2 -> Battery Heater1/2
  Product3/1 -> Battery Heater1/1
  [V_bus] -> Product3/1
  [I_bf] -> Product3/2
  TH0006_flowConfluence4/1 -> Fuel Cell Thermal Mass/2
  Add Constant3/1 -> SC0002_signalRead8/1
  Demux1/1 -> Add Constant3/1
  Saturation1/1 -> Sum2/1
  "Bus Voltage Control 2 "/1(I_fc+ [A]) -> Saturation1/1
  Side Radiator Valve/1 -> [CL4]
  Side Radiator Valve/2 -> TH0016_calculateHeatflow1/2, Radiator & Condenser Assembly/4(CL: (T1,p1,W1))
  Constant/1 -> Side Radiator Valve/1
  TH0006_flowConfluence1/1 -> TH0006_flowConfluence4/2
  TH0006_flowConfluence4/2 -> [SPLIT1]
  [SPLIT2] -> Side Radiator Valve/3
  SC0003_signalWrite10/1 -> Side radiator/3(fan_speed [rpm])
  Constant27/1 -> Side radiator/2(v [m/s])
  [amb] -> Side radiator/1(AMB: (T,p,RH))
  Side radiator/2(CL: (T2,p2,W2)) -> TH0016_calculateHeatflow/1, [CL5]
  [CL1] -> TH0006_flowConfluence4/1
  Side radiator/1(I_fan [A]) -> [I_sideFan2]
  [I_sideFan2] -> Add2/7
  [CL4] -> TH0016_calculateHeatflow/2, Side radiator/4(CL: (T1,p1,W1))
  TH0016_calculateHeatflow/1 -> SC0002_signalRead44/1
  TH0016_calculateHeatflow1/1 -> SC0002_signalRead45/1
  Constant25/1 -> Sum8/1
  Constant21/1 -> Product4/1
  Product4/1 -> SC0002_signalRead21/1, Radiator & Condenser Assembly/3(fan_speed [rpm])
  Constant26/1 -> Product5/1
  Constant28/1 -> Sum12/1
  Sum12/1 -> Product5/2
  Subsystem1/1(cv [-]) -> Sum8/2, Radiator Bypass Valve/1, SC0002_signalRead19/1
  Sum8/1 -> Product4/2
  Constant12/1 -> SC0002_signalRead49/1, Sum13/1
  Sum13/1 -> Gain3/1
  Gain3/1 -> Compressor Speed Controller/1
  SC0003_signalWrite8/1 -> Sum13/2

== system FCHEV_sideRadiator/Bus Voltage Control 1 ==
  V_ref - V_bus [V] : Inport
  PID Controller : slpidlib/PID Controller  Controller=PID  Form=Parallel  TimeDomain=Continuous-time  UseExternalTs=off  SampleTime=-1  IntegratorMethod=Forward Euler  FilterMethod=Forward Euler  ControllerParametersSource=internal  P=1e2  I=1  UseKiTs=off  D=0  N=100  UseFilter=on  TunerSelectOption=Transfer Function Based (PID Tuner App)  ZeroCross=off  InitialConditionSource=internal  InitialConditionForIntegrator=0  InitialConditionForFilter=0  DifferentiatorICPrevScaledInput=0  ExternalReset=none  TrackingMode=off  Kt=1  LimitOutput=on  SatLimitsSource=internal  UpperSaturationLimit=720  LowerSaturationLimit=-360  LinearizeAsGain=on  AntiWindupMode=clamping  Kb=1  LimitIntegrator=off  UpperIntegratorSaturationLimit=inf  LowerIntegratorSaturationLimit=-inf  POutMin=[]  POutMax=[]  IOutMin=[]  IOutMax=[]  DOutMin=[]  DOutMax=[]  NOutMin=[]  NOutMax=[]  SumOutMin=[]  SumOutMax=[]  SaturationOutMin=[]  SaturationOutMax=[]  PParamMin=[]  PParamMax=[]  IParamMin=[]  IParamMax=[]  DParamMin=[]  DParamMax=[]  NParamMin=[]  NParamMax=[]  KbParamMin=[]  KbParamMax=[]  KtParamMin=[]  KtParamMax=[]  KbOutMin=[]  KbOutMax=[]  KtOutMin=[]  KtOutMax=[]  IntegratorOutMin=[]  IntegratorOutMax=[]  FilterOutMin=[]  FilterOutMax=[]  SumI1OutMin=[]  SumI1OutMax=[]  SumI2OutMin=[]  SumI2OutMax=[]  SumI3OutMin=[]  SumI3OutMax=[]  SumI4OutMin=[]  SumI4OutMax=[]  SumDOutMin=[]  SumDOutMax=[]  DifferentiatorOutMin=[]  DifferentiatorOutMax=[]  FilterDiffOutCoefMin=[]  FilterDiffOutCoefMax=[]  ReciprocalOutMin=[]  ReciprocalOutMax=[]  SumDenOutMin=[]  SumDenOutMax=[]  SumNumOutMin=[]  SumNumOutMax=[]  DivideOutMin=[]  DivideOutMax=[]  UdiffTsProdOutMin=[]  UdiffTsProdOutMax=[]  NTsProdOutMin=[]  NTsProdOutMax=[]  UintegralTsProdOutMin=[]  UintegralTsProdOutMax=[]  UngainTsProdOutMin=[]  UngainTsProdOutMax=[]  ClampingZeroOutDataTypeStr=Inherit: Inherit via back propagation  ClampingZeroOutMin=[]  ClampingZeroOutMax=[]  FilterDenConstantOutDataTypeStr=Inherit: Inherit via back propagation  FilterDenConstantOutMin=[]  FilterDenConstantOutMax=[]  PCopyOutDataTypeStr=Inherit: Inherit via back propagation  PCopyOutMin=[]  PCopyOutMax=[]  NCopyOutDataTypeStr=Inherit: Inherit via back propagation  NCopyOutMin=[]  NCopyOutMax=[]  IntegratorContinuousStateAttributes=''  IntegratorStateMustResolveToSignalObject=off  IntegratorRTWStateStorageClass=Auto  FilterContinuousStateAttributes=''  FilterStateMustResolveToSignalObject=off  FilterRTWStateStorageClass=Auto  ParallelPVariant=InternalParameters  IdealPVariant=Disabled  IVariant=InternalParameters  DVariant=InternalParameters  IntegratorVariant=Continuous  SatVariant=Enabled  AWVariant=ContClampingParallel  PCopyVariant=Disabled  TRVariant=Disabled  FdbkBlocksVariant=Forward  IdealPFdbkVariant=Disabled  SatFdbkVariant=Disabled  DerivativeFilterVariant=ContFilter  NVariant=InternalParameters  NCopyVariant=Disabled  FilterICVariant=InternalICsFilter  IntegratorICVariant=InternalICs  ExternalResetVariant=Disabled  TRSumVariant=Passthrough  SumFdbkVariant=Disabled  SumVariant=Sum_PID  TsampFilterVariant=InternalTs  TsampNgainVariant=Passthrough  TsampIntegralVariant=Disabled_SignalSpec  ExternalSaturationOutDataTypeStr=Inherit: Same as second input
  I_bat [-] : Outport
  wires:
  PID Controller/1 -> I_bat [-]/1
  V_ref - V_bus [V]/1 -> PID Controller/1

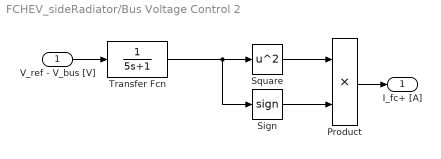
== system FCHEV_sideRadiator/Bus Voltage Control 2  ==
  V_ref - V_bus [V] : Inport
  Product : Product
  Sign : Signum
  Square : Math  Operator=square
  Transfer Fcn : TransferFcn  Denominator=[5 1]
  I_fc+ [A] : Outport
  wires:
  Sign/1 -> Product/2
  Transfer Fcn/1 -> Sign/1, Square/1
  Square/1 -> Product/1
  V_ref - V_bus [V]/1 -> Transfer Fcn/1
  Product/1 -> I_fc+ [A]/1

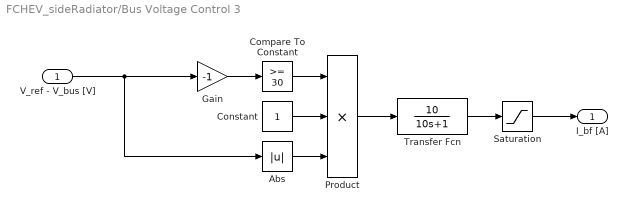
== system FCHEV_sideRadiator/Bus Voltage Control 3 ==
  V_ref - V_bus [V] : Inport
  Abs : Abs  SaturateOnIntegerOverflow=off
  Compare To Constant : simulink/Logic and Bit Operations/Compare To Constant  relop=>=  const=30  OutDataTypeStr=boolean
  Constant : Constant
  Gain : Gain  Gain=-1
  Product : Product  Inputs=3
  Saturation : Saturate  UpperLimit=1000  LowerLimit=0
  Transfer Fcn : TransferFcn  Numerator=[10]  Denominator=[10 1]
  I_bf [A] : Outport
  wires:
  Gain/1 -> Compare To Constant/1
  Transfer Fcn/1 -> Saturation/1
  Compare To Constant/1 -> Product/1
  Product/1 -> Transfer Fcn/1
  V_ref - V_bus [V]/1 -> Abs/1, Gain/1
  Abs/1 -> Product/3
  Constant/1 -> Product/2
  Saturation/1 -> I_bf [A]/1

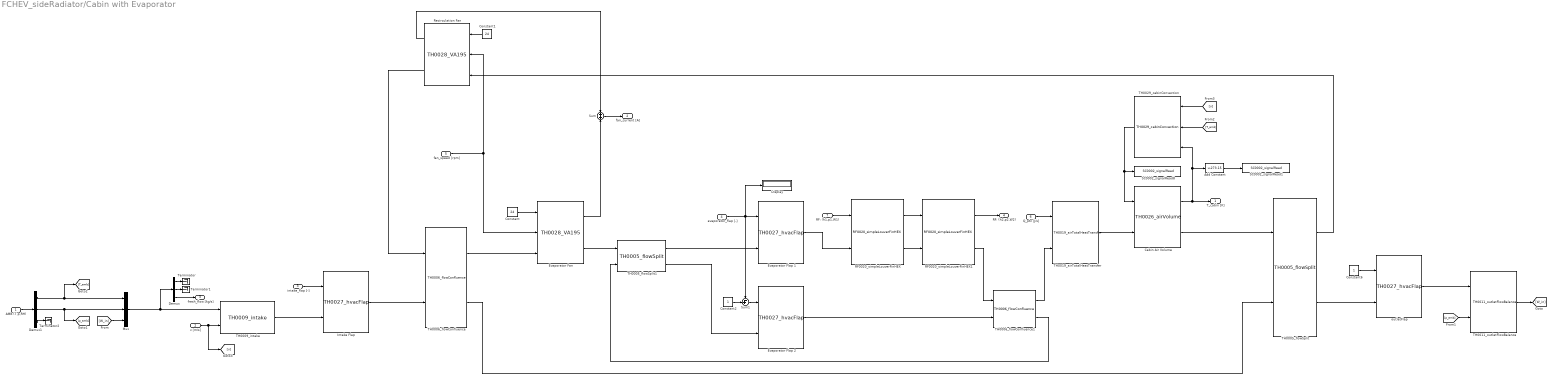
== system FCHEV_sideRadiator/Cabin with Evaporator ==
  AMB (T,p,RH) : Inport
  v [m/s] : Inport  Port=2
  intake_flap [-] : Inport  Port=3
  evaporator_flap [-] : Inport  Port=4
  fan_speed [rpm] : Inport  Port=5
  Q_ptc [J/s] : Inport  Port=6
  RF: (h1,p1,W1) : Inport  Port=7
  Add Constant : Bias  Bias=-273.15  SaturateOnIntegerOverflow=off
  Cabin Air Volume : component_lib/Thermal Systems/TH0026_airVolume  V=4  T0=273.15 + 20
  Constant : Constant  Value=24
  Constant1 : Constant  Value=24
  Constant2 : Constant
  Constant6 : Constant
  Demux : Demux  Outputs=3
  Demux1 : Demux  Outputs=3
  Display : Display
  Evaporator Fan : component_lib/Thermal Systems/TH0028_VA195  n=4
      settings: LibrarySourceBlock=component_lib/Thermal Systems/TH0023_WP120
  Evaporator Flap 1 : component_lib/Thermal Systems/TH0027_hvacFlap  A=0.04  zeta=0.3
  Evaporator Flap 2 : component_lib/Thermal Systems/TH0027_hvacFlap  A=0.04  zeta=0.3
  Intake Flap : component_lib/Thermal Systems/TH0027_hvacFlap  A=0.04  zeta=0.3
  Mux : Mux  Inputs=3
  RF0020_simpleLouverFinHEX : component_lib/Thermal Systems/RF0020_simpleLouverFinHEX  N_tub=20  T_L=0.95*3  T_p=10.15e-3  T_d=16e-3  N_ch=18  a=1.3e-3  b=0.58e-3  L_a=23  F_p=1.4e-3  L_p=1.7e-3  L_l=6.4e-3  H=8.15e-3  d_f=16e-3  F_d=16e-3
  RF0020_simpleLouverFinHEX1 : component_lib/Thermal Systems/RF0020_simpleLouverFinHEX  N_tub=20  T_L=0.95*3  T_p=10.15e-3  T_d=16e-3  N_ch=18  a=1.3e-3  b=0.58e-3  L_a=23  F_p=1.4e-3  L_p=1.7e-3  L_l=6.4e-3  H=8.15e-3  d_f=16e-3  F_d=16e-3
  Recirculation Fan : component_lib/Thermal Systems/TH0028_VA195  n=4
      settings: LibrarySourceBlock=component_lib/Thermal Systems/TH0023_WP120
  SC0002_signalRead1 : component_lib/Data & Control/SC0002_signalRead  SigName=cabinTemperature
  SC0002_signalRead8 : component_lib/Data & Control/SC0002_signalRead  SigName=cabinConvection
  Sum : Sum  Inputs=+|+
  Sum1 : Sum  Inputs=-+|
  TH0005_flowSplit : component_lib/Thermal Systems/TH0005_flowSplit  SystemSampleTime=-1  VariantActivationTime=update diagram  Latency=0  AutoFrameSizeCalculation=off
  TH0005_flowSplit1 : component_lib/Thermal Systems/TH0005_flowSplit  SystemSampleTime=-1  VariantActivationTime=update diagram  Latency=0  AutoFrameSizeCalculation=off
  TH0006_flowConfluence : component_lib/Thermal Systems/TH0006_flowConfluence  gain=0.01
  TH0006_flowConfluence1 : component_lib/Thermal Systems/TH0006_flowConfluence  gain=0.01
  TH0009_intake : component_lib/Thermal Systems/TH0009_intake  zeta=0.1
  TH0011_outletFlowBalance : component_lib/Thermal Systems/TH0011_outletFlowBalance  gain=0.05
  TH0019_airTotalHeatTransfer : component_lib/Thermal Systems/TH0019_airTotalHeatTransfer  T_min=273-40  T_max=273+140
  TH0029_cabinConvection : component_lib/Thermal Systems/TH0029_cabinConvection  A=2
  Terminator : Terminator
  Terminator1 : Terminator
  Terminator2 : Terminator
  outletFlap : component_lib/Thermal Systems/TH0027_hvacFlap  A=0.04  zeta=0.3
  T_cabin [K] : Outport
  fan_current [A] : Outport  Port=2
  fresh_flow [kg/s] : Outport  Port=3
  RF: (h2,p2,W2) : Outport  Port=4
  wires:
  TH0019_airTotalHeatTransfer/1 -> Cabin Air Volume/2
  Q_ptc [J/s]/1 -> TH0019_airTotalHeatTransfer/1
  Add Constant/1 -> SC0002_signalRead1/1
  Demux1/3 -> Terminator2/1
  Demux/2 -> Terminator1/1
  Demux/1 -> Terminator/1
  TH0009_intake/1 -> Intake Flap/2
  Cabin Air Volume/2 -> TH0005_flowSplit/1
  AMB (T,p,RH)/1 -> Demux1/1
  intake_flap [-]/1 -> Intake Flap/1
  Constant/1 -> Evaporator Fan/1
  Intake Flap/1 -> TH0006_flowConfluence/2
  [T_amb] -> TH0029_cabinConvection/2
  v [m/s]/1 -> TH0009_intake/2, [v]
  [v] -> TH0029_cabinConvection/1
  Cabin Air Volume/1 -> T_cabin [K]/1, Add Constant/1, TH0029_cabinConvection/3
  TH0005_flowSplit/2 -> outletFlap/2
  TH0006_flowConfluence/2 -> TH0005_flowSplit/2
  TH0029_cabinConvection/1 -> SC0002_signalRead8/1, Cabin Air Volume/1
  TH0005_flowSplit/1 -> Recirculation Fan/3
  Mux/1 -> Demux/1, TH0009_intake/1
  RF: (h1,p1,W1)/1 -> RF0020_simpleLouverFinHEX/1
  Demux1/2 -> [p_amb], Mux/2
  outletFlap/1 -> TH0011_outletFlowBalance/1
  Demux1/1 -> [T_amb], Mux/1
  [W_in] -> Mux/3
  TH0011_outletFlowBalance/1 -> [W_in]
  Constant6/1 -> outletFlap/1
  [p_amb] -> TH0011_outletFlowBalance/2
  Demux/3 -> fresh_flow [kg/s]/1
  TH0006_flowConfluence/1 -> Evaporator Fan/3
  Recirculation Fan/2 -> TH0006_flowConfluence/1
  Constant1/1 -> Recirculation Fan/1
  fan_speed [rpm]/1 -> Evaporator Fan/2, Recirculation Fan/2
  Evaporator Fan/1 -> Sum/2
  Sum/1 -> fan_current [A]/1
  Recirculation Fan/1 -> Sum/1
  RF0020_simpleLouverFinHEX/1 -> RF0020_simpleLouverFinHEX1/1
  RF0020_simpleLouverFinHEX/2 -> RF0020_simpleLouverFinHEX1/2
  RF0020_simpleLouverFinHEX1/1 -> RF: (h2,p2,W2)/1
  RF0020_simpleLouverFinHEX1/2 -> TH0006_flowConfluence1/1
  Evaporator Fan/2 -> TH0005_flowSplit1/1
  Evaporator Flap 1/1 -> RF0020_simpleLouverFinHEX/2
  evaporator_flap [-]/1 -> Display/1, Sum1/1, Evaporator Flap 1/1
  TH0005_flowSplit1/1 -> Evaporator Flap 1/2
  TH0005_flowSplit1/2 -> Evaporator Flap 2/2
  Constant2/1 -> Sum1/2
  Sum1/1 -> Evaporator Flap 2/1
  TH0006_flowConfluence1/1 -> TH0019_airTotalHeatTransfer/2
  Evaporator Flap 2/1 -> TH0006_flowConfluence1/2
  TH0006_flowConfluence1/2 -> TH0005_flowSplit1/2

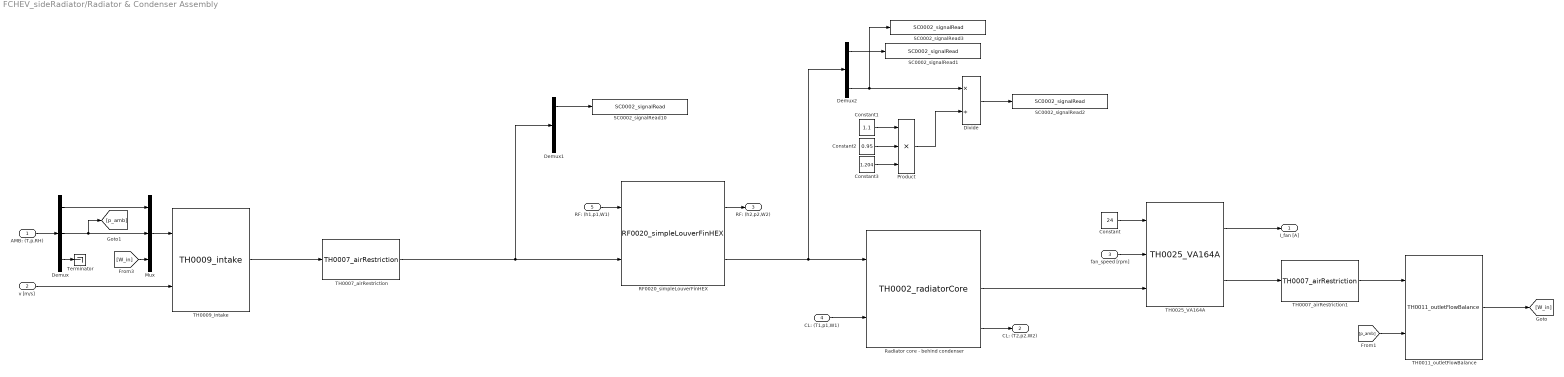
== system FCHEV_sideRadiator/Radiator & Condenser Assembly ==
  AMB: (T,p,RH) : Inport
  v [m/s] : Inport  Port=2
  fan_speed [rpm] : Inport  Port=3
  CL: (T1,p1,W1) : Inport  Port=4
  RF: (h1,p1,W1) : Inport  Port=5
  Constant : Constant  Value=24
  Constant1 : Constant  Value=1.1
  Constant2 : Constant  Value=0.95
  Constant3 : Constant  Value=1.204
  Demux : Demux  Outputs=3
  Demux1 : Demux  Outputs=3
  Demux2 : Demux  Outputs=3
  Divide : Product  Inputs=*/
  Mux : Mux  Inputs=3
  Product : Product  Inputs=3
  RF0020_simpleLouverFinHEX : component_lib/Thermal Systems/RF0020_simpleLouverFinHEX  N_tub=35  T_L=3*0.95  T_p=10.15e-3  T_d=16e-3  N_ch=18  a=1.3e-3  b=0.58e-3  L_a=23  F_p=1.4e-3  L_p=1.7e-3  L_l=6.4e-3  H=8.15e-3  d_f=16e-3  F_d=16e-3
  Radiator core - behind condenser : component_lib/Thermal Systems/TH0002_radiatorCore  HtH=1.1  StS=0.95  radmodel=52 mm
  SC0002_signalRead1 : component_lib/Data & Control/SC0002_signalRead  SigName=airTemperatureAfterCondenser
  SC0002_signalRead10 : component_lib/Data & Control/SC0002_signalRead  SigName=airTemperatureBeforeCondenser
  SC0002_signalRead2 : component_lib/Data & Control/SC0002_signalRead  SigName=radiatorAirVelocity
  SC0002_signalRead3 : component_lib/Data & Control/SC0002_signalRead  SigName=radiatorAirFlow
  TH0007_airRestriction : component_lib/Thermal Systems/TH0007_airRestriction  A=0.5  zeta=0.3
  TH0007_airRestriction1 : component_lib/Thermal Systems/TH0007_airRestriction  A=0.5  zeta=2.4
  TH0009_intake : component_lib/Thermal Systems/TH0009_intake  zeta=0.9
  TH0011_outletFlowBalance : component_lib/Thermal Systems/TH0011_outletFlowBalance  gain=0.05
  TH0025_VA164A : component_lib/Thermal Systems/TH0025_VA164A  n=4
      settings: LibrarySourceBlock=component_lib/Thermal Systems/TH0023_WP120
  Terminator : Terminator
  I_fan [A] : Outport
  CL: (T2,p2,W2) : Outport  Port=2
  RF: (h2,p2,W2) : Outport  Port=3
  wires:
  Constant/1 -> TH0025_VA164A/1
  RF: (h1,p1,W1)/1 -> RF0020_simpleLouverFinHEX/1
  CL: (T1,p1,W1)/1 -> Radiator core - behind condenser/2
  Demux/3 -> Terminator/1
  [W_in] -> Mux/3
  TH0011_outletFlowBalance/1 -> [W_in]
  [p_amb] -> TH0011_outletFlowBalance/2
  Mux/1 -> TH0009_intake/1
  TH0007_airRestriction1/1 -> TH0011_outletFlowBalance/1
  v [m/s]/1 -> TH0009_intake/2
  fan_speed [rpm]/1 -> TH0025_VA164A/2
  AMB: (T,p,RH)/1 -> Demux/1
  Demux/1 -> Mux/1
  Demux/2 -> [p_amb], Mux/2
  RF0020_simpleLouverFinHEX/1 -> RF: (h2,p2,W2)/1
  TH0007_airRestriction/1 -> Demux1/1, RF0020_simpleLouverFinHEX/2
  Radiator core - behind condenser/3 -> CL: (T2,p2,W2)/1
  Demux1/1 -> SC0002_signalRead10/1
  RF0020_simpleLouverFinHEX/2 -> Demux2/1, Radiator core - behind condenser/1
  Demux2/1 -> SC0002_signalRead1/1
  Constant1/1 -> Product/1
  Constant2/1 -> Product/2
  Constant3/1 -> Product/3
  Product/1 -> Divide/2
  Demux2/3 -> SC0002_signalRead3/1, Divide/1
  Divide/1 -> SC0002_signalRead2/1
  TH0025_VA164A/1 -> I_fan [A]/1
  TH0025_VA164A/2 -> TH0007_airRestriction1/1
  TH0009_intake/1 -> TH0007_airRestriction/1
  Radiator core - behind condenser/2 -> TH0025_VA164A/3

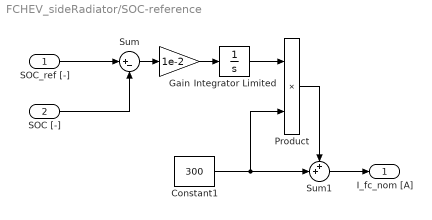
== system FCHEV_sideRadiator/SOC-reference ==
  SOC_ref [-] : Inport
  SOC [-] : Inport  Port=2
  Constant1 : Constant  Value=300
  Gain : Gain  Gain=1e-2
  Integrator Limited : Integrator  LimitOutput=on  UpperSaturationLimit=1  LowerSaturationLimit=-1
  Product : Product
  Sum : Sum  Inputs=|+-
  Sum1 : Sum  Inputs=++|
  I_fc_nom [A] : Outport
  wires:
  Product/1 -> Sum1/1
  Integrator Limited/1 -> Product/1
  Sum1/1 -> I_fc_nom [A]/1
  Constant1/1 -> Sum1/2, Product/2
  Sum/1 -> Gain/1
  SOC [-]/1 -> Sum/2
  Gain/1 -> Integrator Limited/1
  SOC_ref [-]/1 -> Sum/1
